simulink model "Simulink_Model"  (R2020b)
settings: Solver=FixedStepAuto  StartTime=0.0  StopTime=12  FixedStep=1  RelTol=1e-3
values from neighbouring files (symbols this model uses):
  ConstantA = Constants{1}    [Load_config.m]
  ConstantB = Constants{2}    [Load_config.m]
  ConstantC = Constants{3}    [Load_config.m]
  ConstantD = Constants{4}    [Load_config.m]
  ConstantE = Constants{5}    [Load_config.m]
  ConstantF = Constants{6}    [Load_config.m]
  ConstantG = Constants{7}    [Load_config.m]
  ConstantH = Constants{8}    [Load_config.m]
  ConstantI = Constants{9}    [Load_config.m]
  ConstantJ = Constants{18}    [Load_config.m]
  ConstantK = Constants{19}    [Load_config.m]
  ConstantL = Constants{20}    [Load_config.m]
  ConstantM = Constants{21}    [Load_config.m]
  ConstantO = Constants{22}    [Load_config.m]
undefined symbols (not defined in the file or in its folder): A1052, A2, F2, G1052, H2, K1052
libraries: simulink x32, sldvlib x22
(part 3 of 3)

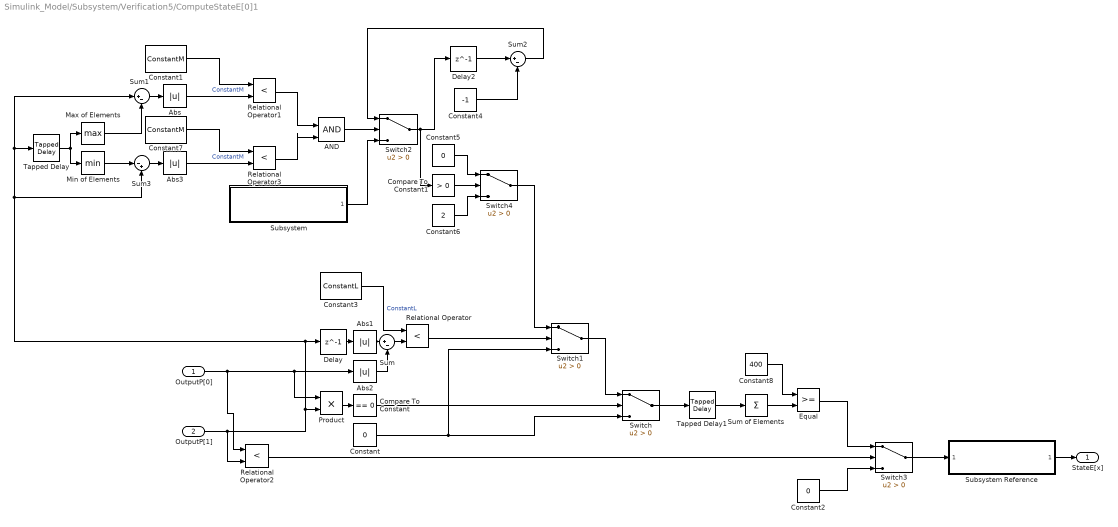
== system Simulink_Model/Subsystem/Verification5/ComputeStateE[0]1 ==
  OutputP[0] : Inport
  OutputP[1] : Inport  Port=2
  AND : Logic  IconShape=distinctive  AllPortsSameDT=off  OutDataTypeStr=boolean
  Abs{,1..3} (4 alike) : Abs
  Compare To Constant : simulink/Logic and Bit Operations/Compare To Constant  relop===  const=0  OutDataTypeStr=boolean
  Compare To Constant1 : simulink/Logic and Bit Operations/Compare To Constant  relop=>  const=0  OutDataTypeStr=boolean
  Constant : Constant  Value=0
  Constant1 : Constant  Value=ConstantM
  Constant2 : Constant  Value=0
  Constant3 : Constant  Value=ConstantL
  Constant4 : Constant  Value=-1
  Constant5 : Constant  Value=0
  Constant6 : Constant  Value=2
  Constant7 : Constant  Value=ConstantM
  Constant8 : Constant  Value=400
  Delay : Delay  DelayLength=1  InitialCondition=0
  Delay2 : Delay  DelayLength=1  InitialCondition=0
  Equal : RelationalOperator  OutDataTypeStr=boolean  RndMeth=Simplest
  Max of Elements : MinMax  Function=max
  Min of Elements : MinMax
  Product : Product
  Relational Operator{,1..3} (4 alike) : RelationalOperator  Operator=<  OutDataTypeStr=boolean  RndMeth=Simplest
  Subsystem : Subsystem  ReferencedSubsystem=CyclesFromSeconds  sec=30
  Subsystem Reference : Subsystem  ReferencedSubsystem=ComputeState
  Sum : Sum  Inputs=|+-
  Sum of Elements : Sum  Inputs=+
  Sum1 : Sum  Inputs=|+-
  Sum2 : Sum  Inputs=|+-
  Sum3 : Sum  Inputs=|-+
  Switch{,1..4} (5 alike) : Switch  Criteria=u2 > Threshold
  Tapped Delay : simulink/Discrete/Tapped Delay  vinit=0.0  samptime=-1  NumDelays=200  DelayOrder=Oldest  includeCurrent=off
  Tapped Delay1 : simulink/Discrete/Tapped Delay  vinit=0.0  samptime=-1  NumDelays=200  DelayOrder=Oldest  includeCurrent=off
  StateE[x] : Outport
  wires:
  OutputP[0]/1 -> Relational Operator2/1, Product/1, Abs2/1
  OutputP[1]/1 -> Relational Operator2/2, Sum3/2, Tapped Delay/1, Sum1/1, Delay/1, Product/2
  Constant/1 -> Switch1/3, Switch/3
  Product/1 -> Compare To Constant/1
  Compare To Constant/1 -> Switch/2
  Constant3/1 -> Relational Operator/1  "ConstantL"
  Sum/1 -> Relational Operator/2
  Relational Operator/1 -> Switch1/2
  Switch1/1 -> Switch/1
  Subsystem Reference/1 -> StateE[x]/1
  Relational Operator2/1 -> Switch3/2
  Constant2/1 -> Switch3/3
  Switch3/1 -> Subsystem Reference/1
  Sum1/1 -> Abs/1
  Abs/1 -> Relational Operator1/2
  Constant1/1 -> Relational Operator1/1  "ConstantM"
  Switch2/1 -> Compare To Constant1/1, Delay2/1
  Delay2/1 -> Sum2/1
  Subsystem/1 -> Switch2/3
  Constant4/1 -> Sum2/2
  Sum2/1 -> Switch2/1
  Compare To Constant1/1 -> Switch4/2
  Constant5/1 -> Switch4/1
  Constant6/1 -> Switch4/3
  Switch4/1 -> Switch1/1
  Delay/1 -> Abs1/1
  Abs1/1 -> Sum/1
  Abs2/1 -> Sum/2
  Tapped Delay/1 -> Min of Elements/1, Max of Elements/1
  Max of Elements/1 -> Sum1/2
  Min of Elements/1 -> Sum3/1
  Sum3/1 -> Abs3/1
  Abs3/1 -> Relational Operator3/2
  Constant7/1 -> Relational Operator3/1  "ConstantM"
  AND/1 -> Switch2/2
  Relational Operator1/1 -> AND/1
  Relational Operator3/1 -> AND/2
  Switch/1 -> Tapped Delay1/1
  Tapped Delay1/1 -> Sum of Elements/1
  Constant8/1 -> Equal/1
  Equal/1 -> Switch3/1
  Sum of Elements/1 -> Equal/2

== system Simulink_Model/Subsystem/Verification6/ComputeStateE[0] ==
  StateE[x] : Inport
  Compare To Constant : simulink/Logic and Bit Operations/Compare To Constant  relop===  const=2  OutDataTypeStr=boolean
  Constant : Constant
  Constant1 : Constant  Value=0
  Constant2 : Constant  Value=2
  Constant5 : Constant  Value=0
  Constant6 : Constant  Value=2
  Delay : Delay  DelayLengthSource=Input port  DelayLength=1  InitialCondition=0
      settings: InputPortMap=u0,p1
  Delay1 : Delay  DelayLength=1  InitialCondition=0
  Delay2 : Delay  DelayLength=1  InitialCondition=0
  OR : Logic  Operator=OR  IconShape=distinctive  AllPortsSameDT=off  OutDataTypeStr=boolean
  Relational Operator : RelationalOperator  Operator=>  OutDataTypeStr=boolean  RndMeth=Simplest
  Relational Operator1 : RelationalOperator  Operator===  OutDataTypeStr=boolean  RndMeth=Simplest
  Subsystem : Subsystem  ReferencedSubsystem=CyclesFromSeconds  sec=0
  Sum : Sum  Inputs=|++
  Sum1 : Sum  Inputs=|+-
  Switch : Switch  Criteria=u2 > Threshold
  Switch2 : Switch  Criteria=u2 > Threshold
  StateF[x] : Outport
  wires:
  StateE[x]/1 -> Compare To Constant/1
  Compare To Constant/1 -> Switch/2
  Constant/1 -> Switch/1
  Constant1/1 -> Switch/3
  Switch/1 -> Sum/1
  Delay/1 -> Sum1/2
  Constant5/1 -> Switch2/3
  Constant6/1 -> Switch2/1
  Switch2/1 -> Delay2/1, StateF[x]/1
  Subsystem/1 -> Delay/2, Relational Operator/2
  Sum/1 -> Sum1/1, Delay/1, Delay1/1
  Sum1/1 -> Relational Operator/1
  Delay1/1 -> Sum/2
  Relational Operator/1 -> OR/1
  Constant2/1 -> Relational Operator1/2
  Delay2/1 -> Relational Operator1/1
  Relational Operator1/1 -> OR/2
  OR/1 -> Switch2/2

== system Simulink_Model/Subsystem/Verification6/ComputeStateE[1] ==
  StateE[x] : Inport
  Compare To Constant : simulink/Logic and Bit Operations/Compare To Constant  relop===  const=2  OutDataTypeStr=boolean
  Constant : Constant
  Constant1 : Constant  Value=0
  Constant2 : Constant  Value=2
  Constant5 : Constant  Value=0
  Constant6 : Constant  Value=2
  Delay : Delay  DelayLengthSource=Input port  DelayLength=1  InitialCondition=0
      settings: InputPortMap=u0,p1
  Delay1 : Delay  DelayLength=1  InitialCondition=0
  Delay2 : Delay  DelayLength=1  InitialCondition=0
  OR : Logic  Operator=OR  IconShape=distinctive  AllPortsSameDT=off  OutDataTypeStr=boolean
  Relational Operator : RelationalOperator  Operator=>  OutDataTypeStr=boolean  RndMeth=Simplest
  Relational Operator1 : RelationalOperator  Operator===  OutDataTypeStr=boolean  RndMeth=Simplest
  Subsystem : Subsystem  ReferencedSubsystem=CyclesFromSeconds  sec=0
  Sum : Sum  Inputs=|++
  Sum1 : Sum  Inputs=|+-
  Switch : Switch  Criteria=u2 > Threshold
  Switch2 : Switch  Criteria=u2 > Threshold
  StateF[x] : Outport
  wires:
  StateE[x]/1 -> Compare To Constant/1
  Compare To Constant/1 -> Switch/2
  Constant/1 -> Switch/1
  Constant1/1 -> Switch/3
  Switch/1 -> Sum/1
  Delay/1 -> Sum1/2
  Constant5/1 -> Switch2/3
  Constant6/1 -> Switch2/1
  Switch2/1 -> Delay2/1, StateF[x]/1
  Subsystem/1 -> Delay/2, Relational Operator/2
  Sum/1 -> Sum1/1, Delay/1, Delay1/1
  Sum1/1 -> Relational Operator/1
  Delay1/1 -> Sum/2
  Relational Operator/1 -> OR/1
  Constant2/1 -> Relational Operator1/2
  Delay2/1 -> Relational Operator1/1
  Relational Operator1/1 -> OR/2
  OR/1 -> Switch2/2
